simulink model "W08_Small_Town_cs"  (R2019a)
settings: Solver=ode5  StartTime=0.0  StopTime=inf  FixedStep=1/60  RelTol=1e-3
PreLoadFcn:
  | mbxruntime.callbacks.PreLoadFcn(bdroot);
PostLoadFcn:
  | mbxruntime.callbacks.PostLoadFcn(bdroot);
InitFcn:
  | mbxruntime.callbacks.InitFcn(bdroot);
StartFcn:
  | mbxruntime.callbacks.StartFcn(bdroot);
StopFcn:
  | mbxruntime.callbacks.StopFcn(bdroot);
model workspace: external: MAT-File .\W08_Small_Town_cs_hws.mat (data not in the file)
undefined symbols (not defined in the file or in its folder): DiscIntNeverNeededParam, InitImageOutputDir, mbxruntime, tabledata, W08_Small_Town_cs_1048b11096256693, W08_Small_Town_cs_2e0572cd922190cb, W08_Small_Town_cs_37c6a902f3501c14, W08_Small_Town_cs_3a6e58e5cc51f637, W08_Small_Town_cs_44a5e1fb92e1ed1e, W08_Small_Town_cs_4cf68a24307ad2e2, W08_Small_Town_cs_4f56285207e9fc6e, W08_Small_Town_cs_6915557c56bccc8a, W08_Small_Town_cs_Audi_A8_Sedan_1_Path_pathUniqueID, W08_Small_Town_cs_b9aebc545fb47dd6, W08_Small_Town_cs_Boy_150_1_Path_pathUniqueID, W08_Small_Town_cs_Boy_150_1_SpeedProfile_speedProfileUniqueID, W08_Small_Town_cs_Citroen_C3_Hatchback_1_Path_pathUniqueID, W08_Small_Town_cs_Male_CyclingCyclist_1_Path_pathUniqueID
libraries: adeye_lib x27, simulink_extras x24, PreScanSimulinkLibrary x2, simulink x2, robotlib x1, PreScanUsefulBlocks x1
(part 2 of 7)

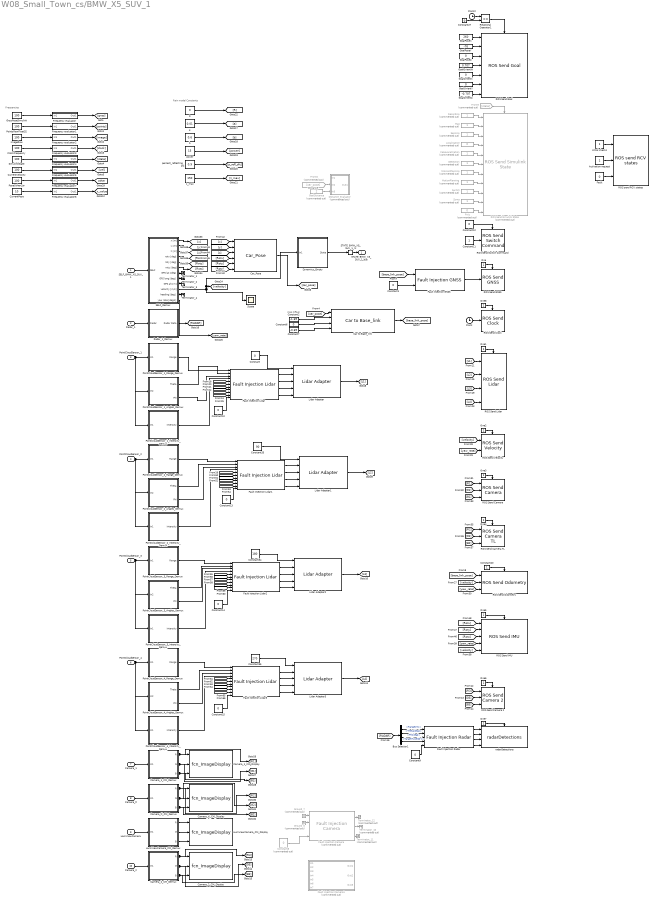
== system W08_Small_Town_cs/BMW_X5_SUV_1 ==
  note: CoG Offset
  note: Distance
  note: Rain model Constants
  note: Frequencies
  SELF_BMW_X5_SUV_1 : Inport  Tag=inport/SelfPort  OutDataTypeStr=Bus: PRESCAN_SELFSENSORDATA  PortDimensions=1  SampleTime=1/60  BusOutputAsStruct=on
  Radar_1 : Inport  Tag=inport/Radar  Port=2  OutDataTypeStr=Bus: PRESCAN_SCANNERSENSOR_MESSAGE  PortDimensions=7  SampleTime=1/20  BusOutputAsStruct=on
  PointCloudSensor_1 : Inport  Tag=inport/PointCloudInport  Port=3  OutDataTypeStr=single  SampleTime=1/20  BusOutputAsStruct=on
  PointCloudSensor_2 : Inport  Tag=inport/PointCloudInport  Port=4  OutDataTypeStr=single  SampleTime=1/20  BusOutputAsStruct=on
  PointCloudSensor_3 : Inport  Tag=inport/PointCloudInport  Port=5  OutDataTypeStr=single  SampleTime=1/20  BusOutputAsStruct=on
  PointCloudSensor_4 : Inport  Tag=inport/PointCloudInport  Port=6  OutDataTypeStr=single  SampleTime=1/20  BusOutputAsStruct=on
  Camera_1 : Inport  Tag=inport/Camera/CameraSensor  Port=7  OutDataTypeStr=uint8  SampleTime=1/20  BusOutputAsStruct=on
  Camera_tl : Inport  Tag=inport/Camera/CameraSensor  Port=8  OutDataTypeStr=uint8  SampleTime=1/20  BusOutputAsStruct=on
  HumViewCamera : Inport  Tag=inport/Camera/CameraSensor  Port=9  OutDataTypeStr=uint8  SampleTime=1/60  BusOutputAsStruct=on
  Camera_2 : Inport  Tag=inport/Camera/CameraSensor  Port=10  OutDataTypeStr=uint8  SampleTime=1/20  BusOutputAsStruct=on
  Activation request : Constant  OutDataTypeStr=Inherit: Inherit via back propagation
  Bus Selector1 : BusSelector  OutputSignals=Range[m],Theta[deg],Phi[deg],TargetTypeID[-]
  Camera_1_CM_Demux : Subsystem  Tag=demux/Camera/Color  mask{SensorName=Camera_1, hres=960, vres=720}
      mask prompts: SensorName "Sensor Name"; hres "Horizontal Resolution"; vres "Vertical Resolution"
      mask Help: eval('openHelp(457)')
      mask Display:
      | fprintf('MONO CAMERA:\n Color\n %s \n %d x %d px',SensorName,hres,vres)
      | port_label('output',1,'R')
      | port_label('output',2,'G')
      | port_label('output',3,'B')
  Camera_1_CM_Display : M-S-Function  Tag=CameraSensor_Color_Display  InitFcn=InitImageOutputDir(gcb);  FunctionName=fcn_ImageDisplay  Parameters=SensorName EnableDisplay EnablePosition DisplayPosition FigureHandle SaveResults BitmapFormat TempOutputDir CameraType DataType  mask(PreScan Color Display Block){SensorName=Camera_1, EnableDisplay=on, EnablePosition=off, DisplayPosition=[10 10 960 720], FigureHandle=567105, SaveResults=off, Format=PNG, TempOutputDir=0, CameraType=Mono, DataType=uint8}
      mask prompts: SensorName "User Specified: Title of Display"; EnableDisplay "Active"; EnablePosition "Set Display window position"; DisplayPosition "Display window position [xpos ypos width height]"; FigureHandle "Unique Handle"; SaveResults "Save results"; TempOutputDir "OutputDir"; CameraType "Camera Type"; DataType "Image Data Type"
      mask help: This block displays the RGB output of a PreScan camera sensor.
      mask init:
      | if EnableDisplay
      |     EnableString='';
      |     EnableColor='gray';
      | else
      |     EnableString='INACTIVE';
      |     EnableColor='red';
      | end
      | switch Format
      |     case 1
      |         BitmapFormat = 'png';
      |     case 2
      |         BitmapFormat = 'bmp';
      |     case 3
      |         BitmapFormat = 'jpg';
      | end 
      | if CameraType==1
      |     CameraTypeName='MONO';
      |     PortNumber=0;
      | else
      |     CameraTypeName='STEREO';
      |     PortNumber=3;
      | end
      settings: CopyFcn=CopyFcnDisplay  DeleteFcn=PreScanBlockDeleteFcn;  ModelCloseFcn=fcn_ImageDisplay_ModelCloseFcn
      mask Help: eval('openHelp(457)')
      mask Callback EnablePosition:
      | MV=get_param(gcb,'MaskVisibilities');
      | if strcmp(get_param(gcb,'EnablePosition'),'on')
      |     MV{4}='on';
      | else
      |     MV{4}='off';
      | end
      | set_param(gcb,'MaskVisibilities',MV);
      | clear MV;
      mask TypeOptions Format: PNG | BMP | JPG
      mask TypeOptions CameraType: Mono | Stereo
      mask TypeOptions DataType: uint8 | single
      mask Display:
      | color(EnableColor);
      | fprintf('%s\n DISPLAY:\n Color \n %s',EnableString,SensorName)
      | port_label('input',1,'R')
      | port_label('input',2,'G')
      | port_label('input',3,'B')
      | port_label('input',PortNumber+1,'R')
      | port_label('input',PortNumber+2,'G')
      | port_label('input',PortNumber+3,'B')
  Camera_2_CM_Demux : Subsystem  Tag=demux/Camera/Color  mask{SensorName=Camera_2, hres=960, vres=720}
      mask prompts: SensorName "Sensor Name"; hres "Horizontal Resolution"; vres "Vertical Resolution"
      mask Help: eval('openHelp(457)')
      mask Display:
      | fprintf('MONO CAMERA:\n Color\n %s \n %d x %d px',SensorName,hres,vres)
      | port_label('output',1,'R')
      | port_label('output',2,'G')
      | port_label('output',3,'B')
  Camera_2_CM_Display : M-S-Function  Tag=CameraSensor_Color_Display  InitFcn=InitImageOutputDir(gcb);  FunctionName=fcn_ImageDisplay  Parameters=SensorName EnableDisplay EnablePosition DisplayPosition FigureHandle SaveResults BitmapFormat TempOutputDir CameraType DataType  mask(PreScan Color Display Block){SensorName=Camera_2, EnableDisplay=on, EnablePosition=off, DisplayPosition=[10 10 960 720], FigureHandle=567108, SaveResults=off, Format=PNG, TempOutputDir=0, CameraType=Mono, DataType=uint8}
      mask prompts: SensorName "User Specified: Title of Display"; EnableDisplay "Active"; EnablePosition "Set Display window position"; DisplayPosition "Display window position [xpos ypos width height]"; FigureHandle "Unique Handle"; SaveResults "Save results"; TempOutputDir "OutputDir"; CameraType "Camera Type"; DataType "Image Data Type"
      mask help: This block displays the RGB output of a PreScan camera sensor.
      mask init: same as W08_Small_Town_cs/BMW_X5_SUV_1/Camera_1_CM_Display
      settings: CopyFcn=CopyFcnDisplay  DeleteFcn=PreScanBlockDeleteFcn;  ModelCloseFcn=fcn_ImageDisplay_ModelCloseFcn
      mask Help: eval('openHelp(457)')
      mask Callback EnablePosition:
      | MV=get_param(gcb,'MaskVisibilities');
      | if strcmp(get_param(gcb,'EnablePosition'),'on')
      |     MV{4}='on';
      | else
      |     MV{4}='off';
      | end
      | set_param(gcb,'MaskVisibilities',MV);
      | clear MV;
      mask TypeOptions Format: PNG | BMP | JPG
      mask TypeOptions CameraType: Mono | Stereo
      mask TypeOptions DataType: uint8 | single
      mask Display:
      | color(EnableColor);
      | fprintf('%s\n DISPLAY:\n Color \n %s',EnableString,SensorName)
      | port_label('input',1,'R')
      | port_label('input',2,'G')
      | port_label('input',3,'B')
      | port_label('input',PortNumber+1,'R')
      | port_label('input',PortNumber+2,'G')
      | port_label('input',PortNumber+3,'B')
  Camera_tl_CM_Demux : Subsystem  Tag=demux/Camera/Color  mask{SensorName=Camera_tl, hres=960, vres=720}
      mask prompts: SensorName "Sensor Name"; hres "Horizontal Resolution"; vres "Vertical Resolution"
      mask Help: eval('openHelp(457)')
      mask Display:
      | fprintf('MONO CAMERA:\n Color\n %s \n %d x %d px',SensorName,hres,vres)
      | port_label('output',1,'R')
      | port_label('output',2,'G')
      | port_label('output',3,'B')
  Camera_tl_CM_Display : M-S-Function  Tag=CameraSensor_Color_Display  InitFcn=InitImageOutputDir(gcb);  FunctionName=fcn_ImageDisplay  Parameters=SensorName EnableDisplay EnablePosition DisplayPosition FigureHandle SaveResults BitmapFormat TempOutputDir CameraType DataType  mask(PreScan Color Display Block){SensorName=Camera_tl, EnableDisplay=on, EnablePosition=off, DisplayPosition=[10 10 960 720], FigureHandle=567106, SaveResults=off, Format=PNG, TempOutputDir=0, CameraType=Mono, DataType=uint8}
      mask prompts: SensorName "User Specified: Title of Display"; EnableDisplay "Active"; EnablePosition "Set Display window position"; DisplayPosition "Display window position [xpos ypos width height]"; FigureHandle "Unique Handle"; SaveResults "Save results"; TempOutputDir "OutputDir"; CameraType "Camera Type"; DataType "Image Data Type"
      mask help: This block displays the RGB output of a PreScan camera sensor.
      mask init: same as W08_Small_Town_cs/BMW_X5_SUV_1/Camera_1_CM_Display
      settings: CopyFcn=CopyFcnDisplay  DeleteFcn=PreScanBlockDeleteFcn;  ModelCloseFcn=fcn_ImageDisplay_ModelCloseFcn
      mask Help: eval('openHelp(457)')
      mask Callback EnablePosition:
      | MV=get_param(gcb,'MaskVisibilities');
      | if strcmp(get_param(gcb,'EnablePosition'),'on')
      |     MV{4}='on';
      | else
      |     MV{4}='off';
      | end
      | set_param(gcb,'MaskVisibilities',MV);
      | clear MV;
      mask TypeOptions Format: PNG | BMP | JPG
      mask TypeOptions CameraType: Mono | Stereo
      mask TypeOptions DataType: uint8 | single
      mask Display:
      | color(EnableColor);
      | fprintf('%s\n DISPLAY:\n Color \n %s',EnableString,SensorName)
      | port_label('input',1,'R')
      | port_label('input',2,'G')
      | port_label('input',3,'B')
      | port_label('input',PortNumber+1,'R')
      | port_label('input',PortNumber+2,'G')
      | port_label('input',PortNumber+3,'B')
  Car to Base_link : adeye_lib/Car to Base_link  SystemSampleTime=-1
  Car_Pose : adeye_lib/Car_Pose  SystemSampleTime=-1
  Clock : Clock
  Clock2 : Clock
  ClockFrequency : Constant  Value=100
  Constant{,10,13..15} (5 alike) : Constant  Value=0  OutDataTypeStr=Inherit: Inherit via back propagation
  Constant1 : Constant  Value=0  OutDataTypeStr=Inherit: Inherit via back propagation  SampleTime=0.05
  Constant11 : Constant  OutDataTypeStr=Inherit: Inherit via back propagation  SampleTime=0.05
  Constant12 : Constant  Value=0  OutDataTypeStr=Inherit: Inherit via back propagation  SampleTime=0.05
  Constant2 : Constant  Value=-1.69
  Constant20 : Constant
  Constant27 : Constant  Value=0
  Constant33 : Constant  Value=90  OutDataTypeStr=Inherit: Inherit via back propagation
  Constant34 : Constant  Value=180  OutDataTypeStr=Inherit: Inherit via back propagation
  Constant35 : Constant  Value=270  OutDataTypeStr=Inherit: Inherit via back propagation
  Constant6 : Constant  Value=0
  Constant7 : Constant  Value=-0.69
  Constant8 : Constant  Commented=on  Value=0
  Constant9 : Constant  Value=0
  CurrentPose : Constant  Value=10
  CurrentVelocity : Constant  Value=100
  Detection : Constant  Commented=on
  Distance_evaluator : Subsystem  Commented=on
  Dynamics_Empty : Subsystem  Tag=Dynamics_Empty
      mask Help: eval('openHelp(202)')
      mask Display: port_label('output', 1, 'State');text(0,0,' Empty\n')
  FakeLocalization : Constant  Commented=on
  Fault : Constant  Value=0  OutDataTypeStr=Inherit: Inherit via back propagation
  Fault Injection Camera : adeye_lib/Fault Injection Camera  Commented=on  idy=200  idx=100  x=100  y=150  R=0  G=0  B=0
  Fault Injection Camera1 : Subsystem  Commented=on
      mask Display:
      | fprintf('Fault inj\n Camera\n')
      | 
      | port_label('input',1,'dx')
      | port_label('input',2,'dy')
      | port_label('input',3,'Error')
      | port_label('input',4,'R')
      | port_label('input',5,'G')
      | port_label('input',6,'B')
      | port_label('input',7,'On/Off')
      | 
      | port_label('output',1,'R')
      | port_label('output',2,'G')
      | port_label('output',3,'B')
  Fault Injection GNSS : adeye_lib/Fault Injection GNSS  v=0.0001  f=20
  Fault Injection Lidar{,1..3} (4 alike) : adeye_lib/Fault Injection Lidar  vr=0.0001  vi=0.0001  f=20  p=225*16
  Fault Injection Radar : adeye_lib/Fault Injection Radar  n=7  vr=1  vt=1  vp=1
  Frequency evaluator : Subsystem
  Frequency evaluator1 : Subsystem
  Frequency evaluator2 : Subsystem
  Frequency evaluator3 : Subsystem
  Frequency evaluator4 : Subsystem
  Frequency evaluator5 : Subsystem
  Frequency evaluator6 : Subsystem
  Frequency evaluator7 : Subsystem
  From6 : From  Commented=on  GotoTag=car_pose
  From9 : From  Commented=on  GotoTag=state
  GnssPoseSimulink : Constant  Value=100
  GoalDistance : Constant  Commented=on  Value=2
  GoalOrientW : Constant  Value=0.707
  GoalOrientX : Constant  Value=0
  GoalOrientY : Constant  Value=0
  GoalOrientZ : Constant  Value=-0.707
  GoalPoseX : Constant  Value=260
  GoalPoseY : Constant  Value=-76
  GoalPoseZ : Constant  Value=0
  Ground_6 : Ground  Commented=on
  Ground_7 : Ground  Commented=on
  HumViewCamera_CM_Demux : Subsystem  Tag=demux/Camera/Color  mask{SensorName=HumViewCamera, hres=1871, vres=1080}
      mask prompts: SensorName "Sensor Name"; hres "Horizontal Resolution"; vres "Vertical Resolution"
      mask Help: eval('openHelp(457)')
      mask Display:
      | fprintf('MONO CAMERA:\n Color\n %s \n %d x %d px',SensorName,hres,vres)
      | port_label('output',1,'R')
      | port_label('output',2,'G')
      | port_label('output',3,'B')
  HumViewCamera_CM_Display : M-S-Function  Tag=CameraSensor_Color_Display  InitFcn=InitImageOutputDir(gcb);  FunctionName=fcn_ImageDisplay  Parameters=SensorName EnableDisplay EnablePosition DisplayPosition FigureHandle SaveResults BitmapFormat TempOutputDir CameraType DataType  mask(PreScan Color Display Block){SensorName=HumViewCamera, EnableDisplay=on, EnablePosition=off, DisplayPosition=[10 10 1871 1080], FigureHandle=567107, SaveResults=off, Format=PNG, TempOutputDir=0, CameraType=Mono, DataType=uint8}
      mask prompts: SensorName "User Specified: Title of Display"; EnableDisplay "Active"; EnablePosition "Set Display window position"; DisplayPosition "Display window position [xpos ypos width height]"; FigureHandle "Unique Handle"; SaveResults "Save results"; TempOutputDir "OutputDir"; CameraType "Camera Type"; DataType "Image Data Type"
      mask help: This block displays the RGB output of a PreScan camera sensor.
      mask init: same as W08_Small_Town_cs/BMW_X5_SUV_1/Camera_1_CM_Display
      settings: CopyFcn=CopyFcnDisplay  DeleteFcn=PreScanBlockDeleteFcn;  ModelCloseFcn=fcn_ImageDisplay_ModelCloseFcn
      mask Help: eval('openHelp(457)')
      mask Callback EnablePosition:
      | MV=get_param(gcb,'MaskVisibilities');
      | if strcmp(get_param(gcb,'EnablePosition'),'on')
      |     MV{4}='on';
      | else
      |     MV{4}='off';
      | end
      | set_param(gcb,'MaskVisibilities',MV);
      | clear MV;
      mask TypeOptions Format: PNG | BMP | JPG
      mask TypeOptions CameraType: Mono | Stereo
      mask TypeOptions DataType: uint8 | single
      mask Display:
      | color(EnableColor);
      | fprintf('%s\n DISPLAY:\n Color \n %s',EnableString,SensorName)
      | port_label('input',1,'R')
      | port_label('input',2,'G')
      | port_label('input',3,'B')
      | port_label('input',PortNumber+1,'R')
      | port_label('input',PortNumber+2,'G')
      | port_label('input',PortNumber+3,'B')
  ImageRaw : Constant  Value=100
  Initial checks : Constant  OutDataTypeStr=Inherit: Inherit via back propagation
  Lidar Adapter{,1..3} (4 alike) : adeye_lib/Lidar Adapter  SystemSampleTime=-1
  Localization : Constant  Commented=on  Value=0
  Map : Constant  Commented=on
  MissionPlanning : Constant  Commented=on
  MotionPlanning : Constant  Commented=on
  One{,1..8} (9 alike) : Constant  OutDataTypeStr=Inherit: Inherit via back propagation
  PointCloudSensor_1_Angles_Demux : Subsystem  Tag=demux/PCS/Angles  mask{SensorName=PointCloudSensor_1, offset=225, hres=225, vres=16}
      mask prompts: SensorName "Sensor Name"; offset "Data Start"; hres "Horizontal Resolution"; vres "Vertical Resolution"
      mask Help: eval('openHelp(6400)')
      mask Display:
      | fprintf('Point Cloud:\n Data\n %s \n %d x %d px',SensorName,hres,vres)
      | port_label('output',1,'Theta')
      | port_label('output',2,'Phi')
  PointCloudSensor_1_Intensity_Demux : Subsystem  Tag=demux/PCS/Intensity  mask{SensorName=PointCloudSensor_1, offset=675, hres=225, vres=16}
      mask prompts: SensorName "Sensor Name"; offset "Data Start"; hres "Horizontal Resolution"; vres "Vertical Resolution"
      mask Help: eval('openHelp(6400)')
      mask Display:
      | fprintf('Point Cloud:\n Data\n %s \n %d x %d px',SensorName,hres,vres)
      | port_label('output',1,'Intensity')
  PointCloudSensor_1_Range_Demux : Subsystem  Tag=demux/PCS/Range  mask{SensorName=PointCloudSensor_1, offset=0, hres=225, vres=16}
      mask prompts: SensorName "Sensor Name"; offset "Data Start"; hres "Horizontal Resolution"; vres "Vertical Resolution"
      mask Help: eval('openHelp(6400)')
      mask Display:
      | fprintf('Point Cloud:\n Data\n %s \n %d x %d px',SensorName,hres,vres)
      | port_label('output',1,'Range')
  PointCloudSensor_2_Angles_Demux : Subsystem  Tag=demux/PCS/Angles  mask{SensorName=PointCloudSensor_2, offset=225, hres=225, vres=16}
      mask prompts: SensorName "Sensor Name"; offset "Data Start"; hres "Horizontal Resolution"; vres "Vertical Resolution"
      mask Help: eval('openHelp(6400)')
      mask Display:
      | fprintf('Point Cloud:\n Data\n %s \n %d x %d px',SensorName,hres,vres)
      | port_label('output',1,'Theta')
      | port_label('output',2,'Phi')
  PointCloudSensor_2_Intensity_Demux : Subsystem  Tag=demux/PCS/Intensity  mask{SensorName=PointCloudSensor_2, offset=675, hres=225, vres=16}
      mask prompts: SensorName "Sensor Name"; offset "Data Start"; hres "Horizontal Resolution"; vres "Vertical Resolution"
      mask Help: eval('openHelp(6400)')
      mask Display:
      | fprintf('Point Cloud:\n Data\n %s \n %d x %d px',SensorName,hres,vres)
      | port_label('output',1,'Intensity')
  PointCloudSensor_2_Range_Demux : Subsystem  Tag=demux/PCS/Range  mask{SensorName=PointCloudSensor_2, offset=0, hres=225, vres=16}
      mask prompts: SensorName "Sensor Name"; offset "Data Start"; hres "Horizontal Resolution"; vres "Vertical Resolution"
      mask Help: eval('openHelp(6400)')
      mask Display:
      | fprintf('Point Cloud:\n Data\n %s \n %d x %d px',SensorName,hres,vres)
      | port_label('output',1,'Range')
  PointCloudSensor_3_Angles_Demux : Subsystem  Tag=demux/PCS/Angles  mask{SensorName=PointCloudSensor_3, offset=225, hres=225, vres=16}
      mask prompts: SensorName "Sensor Name"; offset "Data Start"; hres "Horizontal Resolution"; vres "Vertical Resolution"
      mask Help: eval('openHelp(6400)')
      mask Display:
      | fprintf('Point Cloud:\n Data\n %s \n %d x %d px',SensorName,hres,vres)
      | port_label('output',1,'Theta')
      | port_label('output',2,'Phi')
  PointCloudSensor_3_Intensity_Demux : Subsystem  Tag=demux/PCS/Intensity  mask{SensorName=PointCloudSensor_3, offset=675, hres=225, vres=16}
      mask prompts: SensorName "Sensor Name"; offset "Data Start"; hres "Horizontal Resolution"; vres "Vertical Resolution"
      mask Help: eval('openHelp(6400)')
      mask Display:
      | fprintf('Point Cloud:\n Data\n %s \n %d x %d px',SensorName,hres,vres)
      | port_label('output',1,'Intensity')
  PointCloudSensor_3_Range_Demux : Subsystem  Tag=demux/PCS/Range  mask{SensorName=PointCloudSensor_3, offset=0, hres=225, vres=16}
      mask prompts: SensorName "Sensor Name"; offset "Data Start"; hres "Horizontal Resolution"; vres "Vertical Resolution"
      mask Help: eval('openHelp(6400)')
      mask Display:
      | fprintf('Point Cloud:\n Data\n %s \n %d x %d px',SensorName,hres,vres)
      | port_label('output',1,'Range')
  PointCloudSensor_4_Angles_Demux : Subsystem  Tag=demux/PCS/Angles  mask{SensorName=PointCloudSensor_4, offset=225, hres=225, vres=16}
      mask prompts: SensorName "Sensor Name"; offset "Data Start"; hres "Horizontal Resolution"; vres "Vertical Resolution"
      mask Help: eval('openHelp(6400)')
      mask Display:
      | fprintf('Point Cloud:\n Data\n %s \n %d x %d px',SensorName,hres,vres)
      | port_label('output',1,'Theta')
      | port_label('output',2,'Phi')
  PointCloudSensor_4_Intensity_Demux : Subsystem  Tag=demux/PCS/Intensity  mask{SensorName=PointCloudSensor_4, offset=675, hres=225, vres=16}
      mask prompts: SensorName "Sensor Name"; offset "Data Start"; hres "Horizontal Resolution"; vres "Vertical Resolution"
      mask Help: eval('openHelp(6400)')
      mask Display:
      | fprintf('Point Cloud:\n Data\n %s \n %d x %d px',SensorName,hres,vres)
      | port_label('output',1,'Intensity')
  PointCloudSensor_4_Range_Demux : Subsystem  Tag=demux/PCS/Range  mask{SensorName=PointCloudSensor_4, offset=0, hres=225, vres=16}
      mask prompts: SensorName "Sensor Name"; offset "Data Start"; hres "Horizontal Resolution"; vres "Vertical Resolution"
      mask Help: eval('openHelp(6400)')
      mask Display:
      | fprintf('Point Cloud:\n Data\n %s \n %d x %d px',SensorName,hres,vres)
      | port_label('output',1,'Range')
  PointsRawFloat32 : Constant  Value=100
  PoseOtherCar : Constant  Value=100
  R : Constant  Value=0
  ROS Send Camera : adeye_lib/ROS Send Camera  SystemSampleTime=-1
  ROS Send Camera 2 : adeye_lib/ROS Send Camera 2  SystemSampleTime=-1
  ROS Send Camera TL : adeye_lib/ROS Send Camera TL  SystemSampleTime=-1
  ROS Send Clock : adeye_lib/ROS Send Clock  SystemSampleTime=-1
  ROS Send GNSS : adeye_lib/ROS Send GNSS  SystemSampleTime=-1
  ROS Send Goal : adeye_lib/ROS Send Goal  SystemSampleTime=-1
  ROS Send IMU : adeye_lib/ROS Send IMU  SystemSampleTime=-1
  ROS Send Lidar : adeye_lib/ROS Send Lidar  SystemSampleTime=-1
  ROS Send Odometry : adeye_lib/ROS Send Odometry  SystemSampleTime=-1
  ROS Send Simulink State : adeye_lib/ROS Send Simulink State  Commented=on  SystemSampleTime=-1
  ROS Send Switch Command : adeye_lib/ROS Send Switch Command  SystemSampleTime=-1
  ROS Send Velocity : adeye_lib/ROS Send Velocity  SystemSampleTime=-1
  ROS send RCV states : adeye_lib/ROS send RCV states  SystemSampleTime=-1
  Radar_1_Demux : Subsystem  Tag=demux/Radar  TreatAsAtomicUnit=on  mask(PreScan Demux Block: Radar){MAXMESSAGES=7}
      mask prompts: MAXMESSAGES "Number of Objects"
      mask help:
      | The Radar Sensor is a detailed sensor based on a physical radar
      | model that includes Antenna GAIN Maps (AGM) and atmospheric
      | attenuation.
      |
      | For more information, please click Help.
      mask Help: eval('openHelp(1464)')
      mask Display:
      | port_label('input',1,'Radar')
      | port_label('output',1,'Radar Data')
  Recording : Constant  Commented=on
  Relational Operator1 : RelationalOperator  Operator===  OutDataTypeStr=boolean  RndMeth=Simplest
  Rviz : Constant  Commented=on  Value=0
  SELF_Demux : Subsystem  Tag=demux/SelfPort  mask(PreScan Demux Block:){}
      mask help:
      | The SELF port shows (state) information of the actor itself. The outputs are position in the experiment's axis system and the GPS coordinates, and the object's absolute velocity and compass heading.
      |
      | For more information, please click Help.
      settings: DeleteFcn=PreScanBlockDeleteFcn;
      mask Help: eval('openHelp(462)')
      mask Display:
      | port_label('output',1,'x [m]')
      | port_label('output',2,'y [m]')
      | port_label('output',3,'z [m]','texmode','on')
      | port_label('output',4,'Rotx [deg]','texmode','on')
      | port_label('output',5,'Roty [deg]','texmode','on')
      | port_label('output',6,'Rotz [deg]','texmode','on')
      | port_label('output',7,'GPS lat [deg]','texmode','on')
      | port_label('output',8,'GPS long [deg]','texmode','on')
      | port_label('output',9,'GPS alt [m]','texmode','on')
      | port_label('output',10,'Velocity [m/s]')
      | port_label('output',11,'Heading [deg]')
      | port_label('output',12,'Yaw rate [deg/s]')
  STATE_BMW_X5_SUV_1_rc : RateTransition  Tag=mux_rc/StatePort  OutPortSampleTimeOpt=Inherit
  Scope : Scope
  Sensing : Constant  Commented=on
  SimulinkState : Constant  Value=100
  Ssmp : Constant  Commented=on
  Switch : Constant  Commented=on
  Terminator_{1..4} (4 alike) : Terminator
  Terminator_10 : Terminator  Commented=on
  Terminator_11 : Terminator  Commented=on
  Terminator_12 : Terminator  Commented=on
  a : Constant  Value=0.01
  b : Constant  Value=0.6
  percent_reflecting_sfc : Constant  Value=0.9
  power : Constant  Value=15
  radarDetections : adeye_lib/radarDetections  SystemSampleTime=-1
  z_max : Constant  Value=150
  STATE_BMW_X5_SUV_1_bus : Outport  Tag=outport/StatePort  OutDataTypeStr=Bus: PRESCAN_STATEACTUATORDATA  PortDimensions=1  SampleTime=1/60
  tag scope: other=global, x_value=global
  wires:
  Camera_1_CM_Demux/1(R) -> [R1], Camera_1_CM_Display/1
  Camera_1_CM_Demux/2(G) -> [G1], Camera_1_CM_Display/2
  Camera_1_CM_Demux/3(B) -> [B1], Camera_1_CM_Display/3
  Camera_tl_CM_Demux/1(R) -> [R2], Camera_tl_CM_Display/1
  Camera_tl_CM_Demux/2(G) -> [G2], Camera_tl_CM_Display/2
  Camera_tl_CM_Demux/3(B) -> [B2], Camera_tl_CM_Display/3
  Camera_2_CM_Demux/1(R) -> [R3], Camera_2_CM_Display/1
  Camera_2_CM_Demux/2(G) -> [G3], Camera_2_CM_Display/2
  Camera_2_CM_Demux/3(B) -> [B3], Camera_2_CM_Display/3
  Radar_1_Demux/1(Radar Data) -> [RADAR]
  SELF_Demux/1(x [m]) -> [x]
  SELF_Demux/2(y [m]) -> [y]
  SELF_Demux/3(z [m]) -> [z]
  SELF_Demux/4(rotx [deg]) -> [Rotx]
  SELF_Demux/5(roty [deg]) -> [Roty]
  SELF_Demux/6(rotz [deg]) -> [Rotz]
  SELF_Demux/12(yaw rate [deg/s]) -> [yaw_rate]
  [Roty] -> Car_Pose/5
  [Rotz] -> Car_Pose/6
  [z] -> Car_Pose/3
  [y] -> Car_Pose/2
  [Rotx] -> Car_Pose/4
  [x] -> Car_Pose/1
  PointCloudSensor_1_Intensity_Demux/1(Intensity) -> Fault Injection Lidar/4
  [b] -> Fault Injection Lidar/7
  PointCloudSensor_1_Angles_Demux/2(Phi) -> Fault Injection Lidar/3
  [power] -> Fault Injection Lidar/8
  Fault Injection Lidar/2 -> Lidar Adapter/3
  Lidar Adapter/1 -> [L1]
  Fault Injection Lidar/3 -> Lidar Adapter/4
  Fault Injection Lidar/4 -> Lidar Adapter/5
  Fault Injection Lidar/1 -> Lidar Adapter/2
  [z_max] -> Fault Injection Lidar/10
  [a] -> Fault Injection Lidar/6
  [p_refl_sfc] -> Fault Injection Lidar/9
  Constant/1 -> Lidar Adapter/1
  Constant10/1 -> Fault Injection Lidar/11
  [R] -> Fault Injection Lidar/5
  PointCloudSensor_1_Angles_Demux/1(Theta) -> Fault Injection Lidar/2
  Lidar Adapter1/1 -> [L2]
  Fault Injection Lidar1/4 -> Lidar Adapter1/5
  [power] -> Fault Injection Lidar1/8
  [R] -> Fault Injection Lidar1/5
  [b] -> Fault Injection Lidar1/7
  Fault Injection Lidar1/1 -> Lidar Adapter1/2
  [a] -> Fault Injection Lidar1/6
  Fault Injection Lidar1/3 -> Lidar Adapter1/4
  [p_refl_sfc] -> Fault Injection Lidar1/9
  [z_max] -> Fault Injection Lidar1/10
  Constant13/1 -> Fault Injection Lidar1/11
  Fault Injection Lidar1/2 -> Lidar Adapter1/3
  PointCloudSensor_2_Intensity_Demux/1(Intensity) -> Fault Injection Lidar1/4
  PointCloudSensor_2_Angles_Demux/2(Phi) -> Fault Injection Lidar1/3
  Constant33/1 -> Lidar Adapter1/1
  PointCloudSensor_2_Angles_Demux/1(Theta) -> Fault Injection Lidar1/2
  Lidar Adapter2/1 -> [L3]
  [b] -> Fault Injection Lidar2/7
  Constant14/1 -> Fault Injection Lidar2/11
  Fault Injection Lidar2/3 -> Lidar Adapter2/4
  [a] -> Fault Injection Lidar2/6
  [R] -> Fault Injection Lidar2/5
  [p_refl_sfc] -> Fault Injection Lidar2/9
  Fault Injection Lidar2/1 -> Lidar Adapter2/2
  [z_max] -> Fault Injection Lidar2/10
  Constant34/1 -> Lidar Adapter2/1
  [power] -> Fault Injection Lidar2/8
  PointCloudSensor_3_Angles_Demux/1(Theta) -> Fault Injection Lidar2/2
  Fault Injection Lidar2/2 -> Lidar Adapter2/3
  Fault Injection Lidar2/4 -> Lidar Adapter2/5
  PointCloudSensor_3_Intensity_Demux/1(Intensity) -> Fault Injection Lidar2/4
  PointCloudSensor_3_Angles_Demux/2(Phi) -> Fault Injection Lidar2/3
  Lidar Adapter3/1 -> [L4]
  [p_refl_sfc] -> Fault Injection Lidar3/9
  [R] -> Fault Injection Lidar3/5
  [b] -> Fault Injection Lidar3/7
  Fault Injection Lidar3/3 -> Lidar Adapter3/4
  Constant15/1 -> Fault Injection Lidar3/11
  Fault Injection Lidar3/1 -> Lidar Adapter3/2
  [z_max] -> Fault Injection Lidar3/10
  [power] -> Fault Injection Lidar3/8
  Fault Injection Lidar3/2 -> Lidar Adapter3/3
  [a] -> Fault Injection Lidar3/6
  Constant35/1 -> Lidar Adapter3/1
  PointCloudSensor_4_Angles_Demux/2(Phi) -> Fault Injection Lidar3/3
  PointCloudSensor_4_Intensity_Demux/1(Intensity) -> Fault Injection Lidar3/4
  PointCloudSensor_4_Angles_Demux/1(Theta) -> Fault Injection Lidar3/2
  Fault Injection Lidar3/4 -> Lidar Adapter3/5
  Ground_7/1 -> Fault Injection Camera/1
  ? -> Fault Injection Camera/3
  Fault Injection Camera/3 -> Terminator_11/1
  Fault Injection Camera/2 -> Terminator_10/1
  Ground_6/1 -> Fault Injection Camera/2
  Constant8/1 -> Fault Injection Camera/4
  GoalPoseY/1 -> ROS Send Goal/2
  GoalOrientZ/1 -> ROS Send Goal/7
  GoalPoseZ/1 -> ROS Send Goal/3
  GoalOrientY/1 -> ROS Send Goal/6
  Fault Injection GNSS/1 -> ROS Send GNSS/1
  Car to Base_link/1 -> [base_link_pose]
  GoalOrientW/1 -> ROS Send Goal/4
  GoalPoseX/1 -> ROS Send Goal/1
  Constant11/1 -> ROS Send Switch Command/1
  Constant1/1 -> Fault Injection GNSS/2
  [base_link_pose] -> Fault Injection GNSS/1
  Constant12/1 -> ROS Send Switch Command/Enable
  Relational Operator1/1 -> ROS Send Goal/Enable
  GoalOrientX/1 -> ROS Send Goal/5
  Clock2/1 -> Relational Operator1/1
  Constant27/1 -> Relational Operator1/2
  Constant6/1 -> Car to Base_link/3
  Constant7/1 -> Car to Base_link/4
  Constant2/1 -> Car to Base_link/2
  [car_pose] -> Car to Base_link/1
  power/1 -> [power]
  b/1 -> [b]
  R/1 -> [R]
  z_max/1 -> [z_max]
  a/1 -> [a]
  From6/1 -> Distance_evaluator/2(In2)
  percent_reflecting_sfc/1 -> [p_refl_sfc]
  GoalDistance/1 -> Distance_evaluator/3(In3)
  PointsRawFloat32/1 -> Frequency evaluator1/1(In1)
  ClockFrequency/1 -> Frequency evaluator3/1(In1)
  Frequency evaluator7/1(Out1) -> [other]
  Frequency evaluator2/1(Out1) -> [image]
  Frequency evaluator5/1(Out1) -> [vel]
  CurrentVelocity/1 -> Frequency evaluator5/1(In1)
  PoseOtherCar/1 -> Frequency evaluator7/1(In1)
  Frequency evaluator/1(Out1) -> [gnss]
  CurrentPose/1 -> Frequency evaluator6/1(In1)
  GnssPoseSimulink/1 -> Frequency evaluator/1(In1)
  Frequency evaluator1/1(Out1) -> [points]
  Frequency evaluator4/1(Out1) -> [state]
  Frequency evaluator6/1(Out1) -> [x_value]
  SimulinkState/1 -> Frequency evaluator4/1(In1)
  Frequency evaluator3/1(Out1) -> [clock]
  ImageRaw/1 -> Frequency evaluator2/1(In1)
  Fault Injection Camera/1 -> Terminator_12/1
  Car_Pose/1 -> [car_pose]
  PointCloudSensor_4_Range_Demux/1(Range) -> Fault Injection Lidar3/1
  Rviz/1 -> ROS Send Simulink State/11
  FakeLocalization/1 -> ROS Send Simulink State/5
  Activation request/1 -> ROS send RCV states/2
  Fault/1 -> ROS send RCV states/3
  From9/1 -> ROS Send Simulink State/Enable
  Switch/1 -> ROS Send Simulink State/9
  Localization/1 -> ROS Send Simulink State/4
  Initial checks/1 -> ROS send RCV states/1
  Recording/1 -> ROS Send Simulink State/1
  MotionPlanning/1 -> ROS Send Simulink State/8
  Sensing/1 -> ROS Send Simulink State/3
  Ssmp/1 -> ROS Send Simulink State/10
  Map/1 -> ROS Send Simulink State/2
  MissionPlanning/1 -> ROS Send Simulink State/7
  Detection/1 -> ROS Send Simulink State/6
  Constant20/1 -> ROS Send Odometry/Enable
  [velocity] -> ROS Send IMU/5
  [G3] -> ROS Send Camera 2/2
  Fault Injection Radar/4 -> radarDetections/4
  [yaw_rate] -> ROS Send Odometry/3
  One3/1 -> ROS Send Camera/Enable
  [L1] -> ROS Send Lidar/1
  [G1] -> ROS Send Camera/2
  [G2] -> ROS Send Camera TL/2
  [R2] -> ROS Send Camera TL/1
  [Rotz] -> ROS Send IMU/3
  One2/1 -> ROS Send Velocity/Enable
  Bus Selector1/4 -> Fault Injection Radar/4  "<TargetTypeID[-]>"
  One4/1 -> ROS Send Camera TL/Enable
  One5/1 -> ROS Send IMU/Enable
  One6/1 -> ROS Send Camera 2/Enable
  [yaw_rate] -> ROS Send IMU/4
  [Rotx] -> ROS Send IMU/1
  One1/1 -> ROS Send Lidar/Enable
  [velocity] -> ROS Send Velocity/1
  [R3] -> ROS Send Camera 2/1
  [R1] -> ROS Send Camera/1
  [B3] -> ROS Send Camera 2/3
  [yaw_rate] -> ROS Send Velocity/2
  [base_link_pose] -> ROS Send Odometry/1
  [Roty] -> ROS Send IMU/2
  [velocity] -> ROS Send Odometry/2
  Bus Selector1/2 -> Fault Injection Radar/2  "<Theta[deg]>"
  One7/1 -> radarDetections/Enable
  [L3] -> ROS Send Lidar/3
  [B1] -> ROS Send Camera/3
  Bus Selector1/3 -> Fault Injection Radar/3  "<Phi[deg]>"
  Constant9/1 -> Fault Injection Radar/5
  [L4] -> ROS Send Lidar/4
  Bus Selector1/1 -> Fault Injection Radar/1  "<Range[m]>"
  Fault Injection Radar/2 -> radarDetections/2
  [L2] -> ROS Send Lidar/2
  [RADAR] -> Bus Selector1/1
  Fault Injection Radar/3 -> radarDetections/3
  [B2] -> ROS Send Camera TL/3
  Fault Injection Radar/1 -> radarDetections/1
  Clock/1 -> ROS Send Clock/1
  One8/1 -> ROS Send Clock/Enable
  One/1 -> ROS Send GNSS/Enable
  PointCloudSensor_1_Range_Demux/1(Range) -> Fault Injection Lidar/1
  PointCloudSensor_2_Range_Demux/1(Range) -> Fault Injection Lidar1/1
  PointCloudSensor_3_Range_Demux/1(Range) -> Fault Injection Lidar2/1
  SELF_Demux/10(velocity [m/s]) -> Dynamics_Empty/1(In1), [velocity], Scope/1
  STATE_BMW_X5_SUV_1_rc/1 -> STATE_BMW_X5_SUV_1_bus/1
  SELF_BMW_X5_SUV_1/1 -> SELF_Demux/1(SELF)
  Radar_1/1 -> Radar_1_Demux/1(Radar)
  PointCloudSensor_1/1 -> PointCloudSensor_1_Range_Demux/1(In1), PointCloudSensor_1_Angles_Demux/1(In2), PointCloudSensor_1_Intensity_Demux/1(In1)
  PointCloudSensor_2/1 -> PointCloudSensor_2_Range_Demux/1(In1), PointCloudSensor_2_Angles_Demux/1(In2), PointCloudSensor_2_Intensity_Demux/1(In1)
  PointCloudSensor_3/1 -> PointCloudSensor_3_Range_Demux/1(In1), PointCloudSensor_3_Angles_Demux/1(In2), PointCloudSensor_3_Intensity_Demux/1(In1)
  PointCloudSensor_4/1 -> PointCloudSensor_4_Range_Demux/1(In1), PointCloudSensor_4_Angles_Demux/1(In2), PointCloudSensor_4_Intensity_Demux/1(In1)
  Camera_1/1 -> Camera_1_CM_Demux/1(In1)
  Camera_tl/1 -> Camera_tl_CM_Demux/1(In1)
  HumViewCamera/1 -> HumViewCamera_CM_Demux/1(In1)
  HumViewCamera_CM_Demux/1(R) -> HumViewCamera_CM_Display/1
  HumViewCamera_CM_Demux/2(G) -> HumViewCamera_CM_Display/2
  HumViewCamera_CM_Demux/3(B) -> HumViewCamera_CM_Display/3
  Camera_2/1 -> Camera_2_CM_Demux/1(In1)
  Dynamics_Empty/1(State) -> STATE_BMW_X5_SUV_1_rc/1
  SELF_Demux/7(GPS lat [deg]) -> Terminator_1/1
  SELF_Demux/8(GPS long [deg]) -> Terminator_2/1
  SELF_Demux/9(GPS alt [m]) -> Terminator_3/1
  SELF_Demux/11(heading [deg]) -> Terminator_4/1

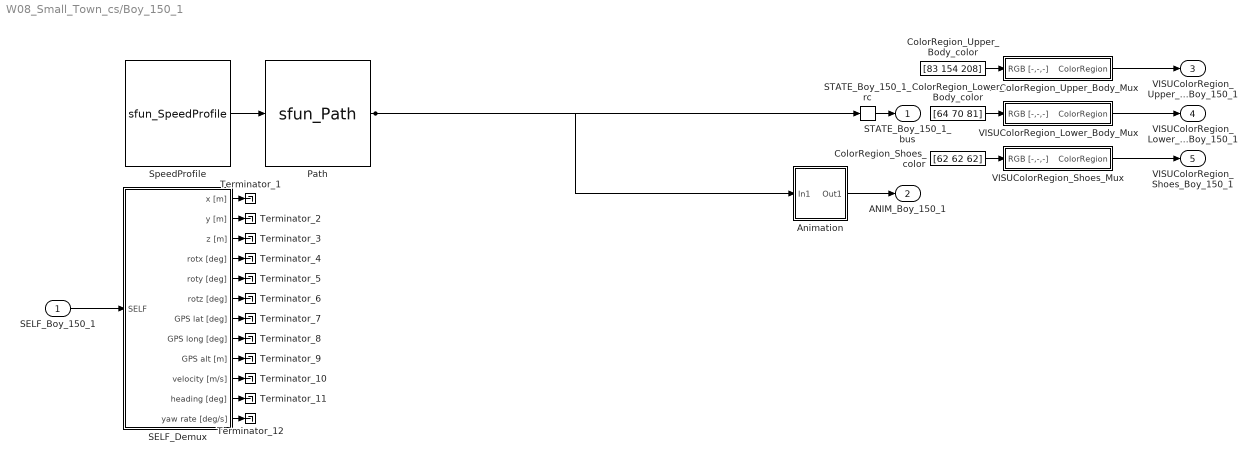
== system W08_Small_Town_cs/Boy_150_1 ==
  SELF_Boy_150_1 : Inport  Tag=inport/SelfPort  OutDataTypeStr=Bus: PRESCAN_SELFSENSORDATA  PortDimensions=1  SampleTime=1/60  BusOutputAsStruct=on
  Animation : Subsystem  Tag=WalkingHumanAnimation  mask(Prescan Conversion Block: Walking Human Animation){TimeStep=1/60}
      mask prompts: TimeStep "Auto-Assigned: Upload Period [s]"
      mask help: The Walking Human Animation block converts the State signal of a human into signals to properly control the animation.
      mask Help: eval('openHelp(239)');
      mask Display: image(imread('HumanAnimated.jpg'))
  ColorRegion_Lower_Body_color : Constant  Tag=VisuLightConst  Value=[64 70 81]
  ColorRegion_Shoes_color : Constant  Tag=VisuLightConst  Value=[62 62 62]
  ColorRegion_Upper_Body_color : Constant  Tag=VisuLightConst  Value=[83 154 208]
  Path : S-Function  Tag=Path  LoadFcn=load('PrescanMotionData.mat')  FunctionName=sfun_Path  Parameters=uniqueID, pathUniqueID, timestep  SFunctionDeploymentMode=off  EnableBusSupport=off  mask(Path){uniqueID=4541, pathUniqueID=W08_Small_Town_cs_Boy_150_1_Path_pathUniqueID, timestep=1/60}
      mask prompts: uniqueID "Object Unique ID"; pathUniqueID "Path Unique ID"; timestep "MATLAB timestep:"
      mask help:
      | The path block outputs the position along a given trajectory.
      |
      | For more information, please click Help.
      mask Help: eval('openHelp(312)')
      mask Display: image(imread('Path.png'))
  SELF_Demux : Subsystem  Tag=demux/SelfPort  mask(PreScan Demux Block:){}
      mask help:
      | The SELF port shows (state) information of the actor itself. The outputs are position in the experiment's axis system and the GPS coordinates, and the object's absolute velocity and compass heading.
      |
      | For more information, please click Help.
      settings: DeleteFcn=PreScanBlockDeleteFcn;
      mask Help: eval('openHelp(462)')
      mask Display:
      | port_label('output',1,'x [m]')
      | port_label('output',2,'y [m]')
      | port_label('output',3,'z [m]','texmode','on')
      | port_label('output',4,'Rotx [deg]','texmode','on')
      | port_label('output',5,'Roty [deg]','texmode','on')
      | port_label('output',6,'Rotz [deg]','texmode','on')
      | port_label('output',7,'GPS lat [deg]','texmode','on')
      | port_label('output',8,'GPS long [deg]','texmode','on')
      | port_label('output',9,'GPS alt [m]','texmode','on')
      | port_label('output',10,'Velocity [m/s]')
      | port_label('output',11,'Heading [deg]')
      | port_label('output',12,'Yaw rate [deg/s]')
  STATE_Boy_150_1_rc : RateTransition  Tag=mux_rc/StatePort  OutPortSampleTimeOpt=Inherit
  SpeedProfile : S-Function  Tag=SpeedProfile  LoadFcn=load('PrescanMotionData.mat')  FunctionName=sfun_SpeedProfile  Parameters=speedProfileUniqueID, timestep  SFunctionDeploymentMode=off  EnableBusSupport=off  mask(SpeedProfile){speedProfileUniqueID=W08_Small_Town_cs_Boy_150_1_SpeedProfile_speedProfileUniqueID, timestep=1/60}
      mask prompts: speedProfileUniqueID "Speed Profile Unique ID"; timestep "MATLAB timestep:"
      mask help:
      | The speed profile block outputs the travelled distance, velocities and acceleration along a given path.
      |
      | For more information, please click Help.
      mask Help: eval('openHelp(312)')
      mask Display: image(imread('SpeedProfile.png'))
  Terminator_{1..12} (12 alike) : Terminator
  VISUColorRegion_Lower_Body_Mux : Subsystem  Tag=mux/MuxColorRegion  LoadFcn=load PrescanColorData  mask(PreScan User Interface: VisuTextureColor){}
      mask help:
      | The VisuTextureColor block provides a way to adapt the color of a vehicle.
      |
      | For more information, please click Help.
      settings: DeleteFcn=PreScanBlockDeleteFcn;
      mask Help: eval('openHelp(230)')
  VISUColorRegion_Shoes_Mux : Subsystem  Tag=mux/MuxColorRegion  LoadFcn=load PrescanColorData  mask(PreScan User Interface: VisuTextureColor){}
      mask help:
      | The VisuTextureColor block provides a way to adapt the color of a vehicle.
      |
      | For more information, please click Help.
      settings: DeleteFcn=PreScanBlockDeleteFcn;
      mask Help: eval('openHelp(230)')
  VISUColorRegion_Upper_Body_Mux : Subsystem  Tag=mux/MuxColorRegion  LoadFcn=load PrescanColorData  mask(PreScan User Interface: VisuTextureColor){}
      mask help:
      | The VisuTextureColor block provides a way to adapt the color of a vehicle.
      |
      | For more information, please click Help.
      settings: DeleteFcn=PreScanBlockDeleteFcn;
      mask Help: eval('openHelp(230)')
  STATE_Boy_150_1_bus : Outport  Tag=outport/StatePort  OutDataTypeStr=Bus: PRESCAN_STATEACTUATORDATA  PortDimensions=1  SampleTime=1/60
  ANIM_Boy_150_1 : Outport  Tag=outport/AnimationOutport  Port=2  OutDataTypeStr=Bus: PRESCAN_ANIMACTUATORDATA  PortDimensions=1  SampleTime=1/60
  VISUColorRegion_Upper_Body_Boy_150_1 : Outport  Tag=outport/ColorRegion  Port=3  OutDataTypeStr=Bus: PRESCAN_COLOR_DATA  PortDimensions=1  SampleTime=1/60
  VISUColorRegion_Lower_Body_Boy_150_1 : Outport  Tag=outport/ColorRegion  Port=4  OutDataTypeStr=Bus: PRESCAN_COLOR_DATA  PortDimensions=1  SampleTime=1/60
  VISUColorRegion_Shoes_Boy_150_1 : Outport  Tag=outport/ColorRegion  Port=5  OutDataTypeStr=Bus: PRESCAN_COLOR_DATA  PortDimensions=1  SampleTime=1/60
  wires:
  STATE_Boy_150_1_rc/1 -> STATE_Boy_150_1_bus/1
  Animation/1(Out1) -> ANIM_Boy_150_1/1
  SpeedProfile/1 -> Path/1
  Path/1 -> STATE_Boy_150_1_rc/1, Animation/1(In1)
  SELF_Boy_150_1/1 -> SELF_Demux/1(SELF)
  VISUColorRegion_Upper_Body_Mux/1(ColorRegion) -> VISUColorRegion_Upper_Body_Boy_150_1/1
  ColorRegion_Upper_Body_color/1 -> VISUColorRegion_Upper_Body_Mux/1(RGB [-,-,-])
  VISUColorRegion_Lower_Body_Mux/1(ColorRegion) -> VISUColorRegion_Lower_Body_Boy_150_1/1
  ColorRegion_Lower_Body_color/1 -> VISUColorRegion_Lower_Body_Mux/1(RGB [-,-,-])
  VISUColorRegion_Shoes_Mux/1(ColorRegion) -> VISUColorRegion_Shoes_Boy_150_1/1
  ColorRegion_Shoes_color/1 -> VISUColorRegion_Shoes_Mux/1(RGB [-,-,-])
  SELF_Demux/1(x [m]) -> Terminator_1/1
  SELF_Demux/2(y [m]) -> Terminator_2/1
  SELF_Demux/3(z [m]) -> Terminator_3/1
  SELF_Demux/4(rotx [deg]) -> Terminator_4/1
  SELF_Demux/5(roty [deg]) -> Terminator_5/1
  SELF_Demux/6(rotz [deg]) -> Terminator_6/1
  SELF_Demux/7(GPS lat [deg]) -> Terminator_7/1
  SELF_Demux/8(GPS long [deg]) -> Terminator_8/1
  SELF_Demux/9(GPS alt [m]) -> Terminator_9/1
  SELF_Demux/10(velocity [m/s]) -> Terminator_10/1
  SELF_Demux/11(heading [deg]) -> Terminator_11/1
  SELF_Demux/12(yaw rate [deg/s]) -> Terminator_12/1

== system W08_Small_Town_cs/Camera_1 ==
  Sensor : S-Function  FunctionName=sfun_Camera  Parameters=sensorID, dataWidth, dataHeight, channelsPerImage, numberOfImages, timestep  SFunctionDeploymentMode=off  EnableBusSupport=off  mask(PreScan Source Block: Camera Sensor){sensorID=5676, dataWidth=720, dataHeight=2880, channelsPerImage=3, numberOfImages=1, timestep=1/20}
      mask prompts: sensorID "Sensor ID"; dataWidth "Data width"; dataHeight "Data Height"; channelsPerImage "Channels per image"; numberOfImages "Number of images"; timestep "MATLAB timestep:"
      mask help: The Camera Sensor provides a color or monochrome image.
      mask Help: eval('openHelp(457)')
      mask Display: image(imread('CameraSensor.png'))
  Camera_1 : Outport  Tag=outport/Camera/CameraSensor  OutDataTypeStr=uint8  SampleTime=1/20
  wires:
  Sensor/1 -> Camera_1/1

== system W08_Small_Town_cs/Camera_2 ==
  Sensor : S-Function  FunctionName=sfun_Camera  Parameters=sensorID, dataWidth, dataHeight, channelsPerImage, numberOfImages, timestep  SFunctionDeploymentMode=off  EnableBusSupport=off  mask(PreScan Source Block: Camera Sensor){sensorID=5680, dataWidth=720, dataHeight=2880, channelsPerImage=3, numberOfImages=1, timestep=1/20}
      mask prompts: sensorID "Sensor ID"; dataWidth "Data width"; dataHeight "Data Height"; channelsPerImage "Channels per image"; numberOfImages "Number of images"; timestep "MATLAB timestep:"
      mask help: The Camera Sensor provides a color or monochrome image.
      mask Help: eval('openHelp(457)')
      mask Display: image(imread('CameraSensor.png'))
  Camera_2 : Outport  Tag=outport/Camera/CameraSensor  OutDataTypeStr=uint8  SampleTime=1/20
  wires:
  Sensor/1 -> Camera_2/1

== system W08_Small_Town_cs/Camera_tl ==
  Sensor : S-Function  FunctionName=sfun_Camera  Parameters=sensorID, dataWidth, dataHeight, channelsPerImage, numberOfImages, timestep  SFunctionDeploymentMode=off  EnableBusSupport=off  mask(PreScan Source Block: Camera Sensor){sensorID=5677, dataWidth=720, dataHeight=2880, channelsPerImage=3, numberOfImages=1, timestep=1/20}
      mask prompts: sensorID "Sensor ID"; dataWidth "Data width"; dataHeight "Data Height"; channelsPerImage "Channels per image"; numberOfImages "Number of images"; timestep "MATLAB timestep:"
      mask help: The Camera Sensor provides a color or monochrome image.
      mask Help: eval('openHelp(457)')
      mask Display: image(imread('CameraSensor.png'))
  Camera_tl : Outport  Tag=outport/Camera/CameraSensor  OutDataTypeStr=uint8  SampleTime=1/20
  wires:
  Sensor/1 -> Camera_tl/1

== system W08_Small_Town_cs/Citroen_C3_Hatchback_1 ==
  SELF_Citroen_C3_Hatchback_1 : Inport  Tag=inport/SelfPort  OutDataTypeStr=Bus: PRESCAN_SELFSENSORDATA  PortDimensions=1  SampleTime=1/60  BusOutputAsStruct=on
  Path : S-Function  Tag=Path  LoadFcn=load('PrescanMotionData.mat')  FunctionName=sfun_Path  Parameters=uniqueID, pathUniqueID, timestep  SFunctionDeploymentMode=off  EnableBusSupport=off  mask(Path){uniqueID=4537, pathUniqueID=W08_Small_Town_cs_Citroen_C3_Hatchback_1_Path_pathUniqueID, timestep=1/60}
      mask prompts: uniqueID "Object Unique ID"; pathUniqueID "Path Unique ID"; timestep "MATLAB timestep:"
      mask help:
      | The path block outputs the position along a given trajectory.
      |
      | For more information, please click Help.
      mask Help: eval('openHelp(312)')
      mask Display: image(imread('Path.png'))
  SELF_Demux : Subsystem  Tag=demux/SelfPort  mask(PreScan Demux Block:){}
      mask help:
      | The SELF port shows (state) information of the actor itself. The outputs are position in the experiment's axis system and the GPS coordinates, and the object's absolute velocity and compass heading.
      |
      | For more information, please click Help.
      settings: DeleteFcn=PreScanBlockDeleteFcn;
      mask Help: eval('openHelp(462)')
      mask Display:
      | port_label('output',1,'x [m]')
      | port_label('output',2,'y [m]')
      | port_label('output',3,'z [m]','texmode','on')
      | port_label('output',4,'Rotx [deg]','texmode','on')
      | port_label('output',5,'Roty [deg]','texmode','on')
      | port_label('output',6,'Rotz [deg]','texmode','on')
      | port_label('output',7,'GPS lat [deg]','texmode','on')
      | port_label('output',8,'GPS long [deg]','texmode','on')
      | port_label('output',9,'GPS alt [m]','texmode','on')
      | port_label('output',10,'Velocity [m/s]')
      | port_label('output',11,'Heading [deg]')
      | port_label('output',12,'Yaw rate [deg/s]')
  STATE_Citroen_C3_Hatchback_1_rc : RateTransition  Tag=mux_rc/StatePort  OutPortSampleTimeOpt=Inherit
  SpeedProfile : S-Function  Tag=SpeedProfile  LoadFcn=load('PrescanMotionData.mat')  FunctionName=sfun_SpeedProfile  Parameters=speedProfileUniqueID, timestep  SFunctionDeploymentMode=off  EnableBusSupport=off  mask(SpeedProfile){speedProfileUniqueID=W08_Small_Town_cs_4f56285207e9fc6e, timestep=1/60}
      mask prompts: speedProfileUniqueID "Speed Profile Unique ID"; timestep "MATLAB timestep:"
      mask help:
      | The speed profile block outputs the travelled distance, velocities and acceleration along a given path.
      |
      | For more information, please click Help.
      mask Help: eval('openHelp(312)')
      mask Display: image(imread('SpeedProfile.png'))
  Terminator_{1..12} (12 alike) : Terminator
  STATE_Citroen_C3_Hatchback_1_bus : Outport  Tag=outport/StatePort  OutDataTypeStr=Bus: PRESCAN_STATEACTUATORDATA  PortDimensions=1  SampleTime=1/60
  wires:
  STATE_Citroen_C3_Hatchback_1_rc/1 -> STATE_Citroen_C3_Hatchback_1_bus/1
  SpeedProfile/1 -> Path/1
  Path/1 -> STATE_Citroen_C3_Hatchback_1_rc/1
  SELF_Citroen_C3_Hatchback_1/1 -> SELF_Demux/1(SELF)
  SELF_Demux/1(x [m]) -> Terminator_1/1
  SELF_Demux/2(y [m]) -> Terminator_2/1
  SELF_Demux/3(z [m]) -> Terminator_3/1
  SELF_Demux/4(rotx [deg]) -> Terminator_4/1
  SELF_Demux/5(roty [deg]) -> Terminator_5/1
  SELF_Demux/6(rotz [deg]) -> Terminator_6/1
  SELF_Demux/7(GPS lat [deg]) -> Terminator_7/1
  SELF_Demux/8(GPS long [deg]) -> Terminator_8/1
  SELF_Demux/9(GPS alt [m]) -> Terminator_9/1
  SELF_Demux/10(velocity [m/s]) -> Terminator_10/1
  SELF_Demux/11(heading [deg]) -> Terminator_11/1
  SELF_Demux/12(yaw rate [deg/s]) -> Terminator_12/1
